simulink model "Pole_Placement_vs_Dual_System"  (R2023b)
settings: Solver=VariableStepAuto  StartTime=0.0  StopTime=5  MaxStep=1e-3  RelTol=1e-3
values from neighbouring files (symbols this model uses):
  A = [1 4;2 1]    [Compensator_Parameters.m]
  B = [1;1]    [Compensator_Parameters.m]
  C = [0 1]    [Compensator_Parameters.m]
  L = acker(A',C',[-1 -2])'    [Compensator_Parameters.m]
  Lop = Lt'    [Compensator_Parameters.m]
  N = 1/dcgain(A-B*K,B,C,0)    [Compensator_Parameters.m]
undefined symbols (not defined in the file or in its folder): K
settings Model: Creator=Usuario  LastModifiedBy=JHL
settings SolverCC: AlgebraicLoopSolver=TrustRegion
settings DataIOCC: ReturnWorkspaceOutputs=off
settings DebuggingCC: UnconnectedInputMsg=warning  UnconnectedOutputMsg=warning  UnconnectedLineMsg=warning  ArithmeticOperatorsInVariantConditions=warning
settings ModelReferenceCC: EnableRefExpFcnMdlSchedulingChecks=on
settings SFSimCC: SimUseLocalCustomCode=off  CustomCodeUndefinedFunction=UseInterfaceOnly
settings RTWCC: RTWUseLocalCustomCode=off

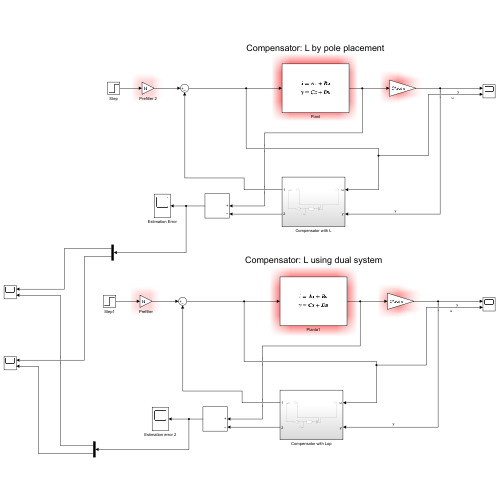
[thumbnail: Simulink's stored preview of the top-level diagram]
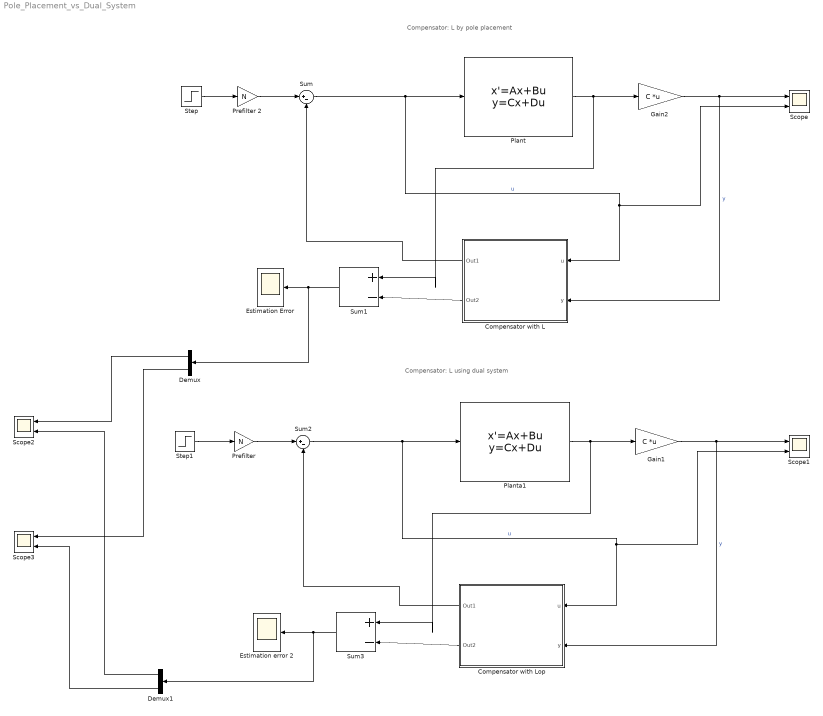
== system Pole_Placement_vs_Dual_System ==
  note: Compensator: L by pole placement
  note: Compensator: L using dual system
  Compensator with L : Subsystem
  Compensator with Lop : Subsystem
  Demux : Demux  Outputs=2
  Demux1 : Demux  Outputs=2
  Estimation Error : Scope
  Estimation error 2 : Scope
  Gain1 : Gain  Gain=C  Multiplication=Matrix(K*u) (u vector)
  Gain2 : Gain  Gain=C  Multiplication=Matrix(K*u) (u vector)
  Plant : StateSpace  A=A  B=B  C=eye(2)  D=zeros(2,1)  InitialCondition=0
  Planta1 : StateSpace  A=A  B=B  C=eye(2)  D=zeros(2,1)  InitialCondition=0
  Prefilter : Gain  Gain=N
  Prefilter 2 : Gain  Gain=N
  Scope{,1..3} (4 alike) : Scope  NumInputPorts=2
  Step : Step  SampleTime=0
  Step1 : Step  SampleTime=0
  Sum{,1..3} (4 alike) : Sum  Inputs=|+-
  wires:
  Plant/1 -> Sum1/1, Gain2/1
  Gain2/1 -> Compensator with L/2(y), Scope/1  "y"
  Sum/1 -> Scope/2, Compensator with L/1(u), Plant/1  "u"
  Prefilter 2/1 -> Sum/1
  Step/1 -> Prefilter 2/1
  Compensator with L/1(Out1) -> Sum/2
  Compensator with L/2(Out2) -> Sum1/2
  Sum1/1 -> Demux/1, Estimation Error/1
  Compensator with Lop/2(Out2) -> Sum3/2
  Sum3/1 -> Demux1/1, Estimation error 2/1
  Sum2/1 -> Scope1/2, Compensator with Lop/1(u), Planta1/1  "u"
  Compensator with Lop/1(Out1) -> Sum2/2
  Gain1/1 -> Compensator with Lop/2(y), Scope1/1  "y"
  Planta1/1 -> Sum3/1, Gain1/1
  Step1/1 -> Prefilter/1
  Prefilter/1 -> Sum2/1
  Demux/1 -> Scope2/1
  Demux1/1 -> Scope2/2
  Demux/2 -> Scope3/1
  Demux1/2 -> Scope3/2

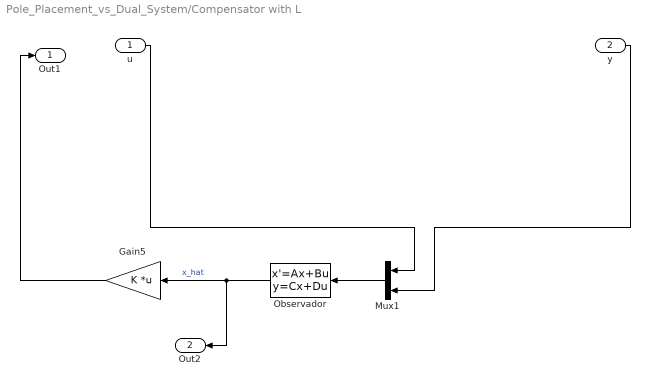
== system Pole_Placement_vs_Dual_System/Compensator with L ==
  u : Inport
  y : Inport  Port=2
  Gain5 : Gain  Gain=K  Multiplication=Matrix(K*u) (u vector)
  Mux1 : Mux  Inputs=2
  Observador : StateSpace  A=A-L*C  B=[B L]  C=eye(2)  D=zeros(2,2)  InitialCondition=0
  Out1 : Outport  VectorParamsAs1DForOutWhenUnconnected=off
  Out2 : Outport  Port=2  VectorParamsAs1DForOutWhenUnconnected=off
  wires:
  Mux1/1 -> Observador/1
  Observador/1 -> Out2/1, Gain5/1  "x_hat"
  y/1 -> Mux1/2
  u/1 -> Mux1/1
  Gain5/1 -> Out1/1

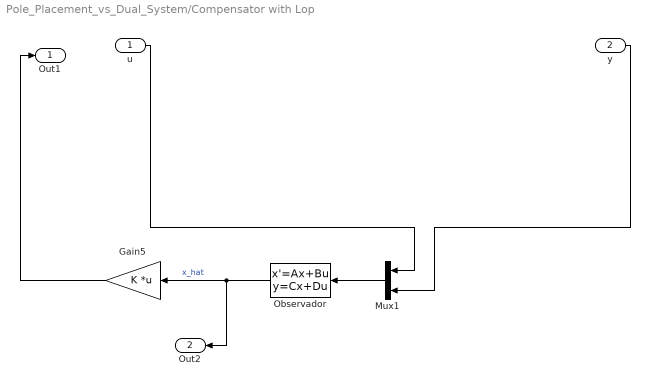
== system Pole_Placement_vs_Dual_System/Compensator with Lop ==
  u : Inport
  y : Inport  Port=2
  Gain5 : Gain  Gain=K  Multiplication=Matrix(K*u) (u vector)
  Mux1 : Mux  Inputs=2
  Observador : StateSpace  A=A-Lop*C  B=[B Lop]  C=eye(2)  D=zeros(2,2)  InitialCondition=0
  Out1 : Outport  VectorParamsAs1DForOutWhenUnconnected=off
  Out2 : Outport  Port=2  VectorParamsAs1DForOutWhenUnconnected=off
  wires:
  Mux1/1 -> Observador/1
  Observador/1 -> Out2/1, Gain5/1  "x_hat"
  y/1 -> Mux1/2
  u/1 -> Mux1/1
  Gain5/1 -> Out1/1
